simulink model "SPGF_FSK_0000_R2022b"  (R2022b)
settings: Solver=ode4  StartTime=0.0  StopTime=1.4  FixedStep=50e-6/50  RelTol=1e-3  EnableMultiTasking=on
undefined symbols (not defined in the file): D11, Delta
libraries: spsSeriesRLCBranchLib x1646, spsGroundLib x360, spsStairGeneratorLib x147, spsIdealSwitchLib x145, spsCurrentMeasurementLib x145, spsUniversalBridgeLib x76, spsThreePhaseSeriesRLCLoadLib x57, simulink x45, spsBistableLib x36, spsSequenceAnalyzerLib x31, spsThreePhaseParallelRLCLoadLib x20, spsThreePhaseTransformerTwoWindingsLib x20
(part 4 of 40)

== system SPGF_FSK_0000_R2022b/K6 ==
  fault : Subsystem  mask(Single Phase-to-Ground Fault){FaultA=on, FaultB=off, FaultC=off, FaultResistance=0.0001, GroundResistance=1e-03, SnubberResistance=1e6, SnubberCapacitance=inf, TransitionTimes=[0.2 0.8], InitialPhaseCtrl=off, Freq=50, Units=degrees, FaultDelayDeg=0, FaultDelayRad=0, FaultDelaySec=0, TheoryOfArc=None, WaitTime=0.008, TypeOfArcIgnVoltage=Stair Pattern with Ramp, ArcVoltage=6000, PulseArcVoltage=[6000 600], DurPulseArcVoltage=0.2, SwitchArcVoltage=[6000 600 5000 400], DurArcVoltage=[0.1 0.2 0.1 0.2], EndArcVoltage=[7000 200 5000 900], LimitArcNum=off, ArcingNumber=1, AddTimeDelay=off, TimeDelay=[0 0.1 0.2 ], EnableFilter=off, FreqFilter=200, FilterReturnTime=1e-3, Inter=off, TypeOfPause=None, NoiseSampleTime=0.04, NoiseSeed=23345, PulsePeriod=0.2, PulseWidth=20, PhaseDelay=0, SwitchTimes=[1 1.01 1.2 1.4]}
      mask prompts: FaultA "Phase A"; FaultB "Phase B"; FaultC "Phase C"; FaultResistance "Fault resistance Ron (ohms) :"; GroundResistance "Ground resistance Rg (ohms) :"; SnubberResistance "Snubbers resistance Rp (ohms) :"; SnubberCapacitance "Snubbers capacitance Cp (F) :"; TransitionTimes "Transition times (s) :"; InitialPhaseCtrl "Enable voltage zero crossing control"; Freq "Fundumental frequency (Hz) :"; Units "Units for fault delay"; FaultDelayDeg "Fault delay (Units) :"; FaultDelayRad "Fault delay (Units) :"; FaultDelaySec "Fault delay (Units) :"; TheoryOfArc "Theory of the arcing ground"; WaitTime "Wait time after the arcing (sec):"; TypeOfArcIgnVoltage "Type of Arc Ignition Voltage"; ArcVoltage "Voltage of the arcing (V) :"; PulseArcVoltage "Voltage of the arcing (V) :"; DurPulseArcVoltage "Duration of pulse (sec) :"; SwitchArcVoltage "Voltage of the arcing (V) :"; DurArcVoltage "Duration of Voltage Arc (sec) :"; EndArcVoltage "Voltage of the arcing at the end of each range (V) :"; LimitArcNum "Limit number of arcing [N] :"; ArcingNumber "Number of uprising arcing"; AddTimeDelay "Add time delay :"; TimeDelay "Time delay between arc (sec) [1xN] :"; EnableFilter "Enable lowpass filter"; FreqFilter "Natural frequency of lowpass filter (Hz) [120-250]:"; FilterReturnTime "Filter return time (sec):"; Inter "Interrupt only arc striking"; TypeOfPause "Add pause in the arcing ground"; NoiseSampleTime "Sample time of white noise (s) :"; NoiseSeed "Seed of white noise"; PulsePeriod "Period of pulses (s) :"; PulseWidth "Width of pulse (% of period) :"; PhaseDelay "Phase delay (sec) :"; SwitchTimes "Switch times (sec) [1,0,1,0...] :"
      mask init: same as SPGF_FSK_0000_R2022b/K2/fault
      settings: CloseFcn=|
      | en = get_param(gcb,'MaskEnables');
      | set_param(gcb,'MaskEnables',en)
      | clear enab en;
      settings: MoveFcn=|
      | en = get_param(gcb,'MaskEnables');
      | set_param(gcb,'MaskEnables',en)
      | clear enab en;
      mask Callback FaultA:
      | maskObj = Simulink.Mask.get(gcb);
      |     enab = get_param(gcb,'FaultA');
      |     if strcmp(enab,'on')
      |         maskObj.getParameter('FaultB').Enabled = 'off';
      |         maskObj.getParameter('FaultC').Enabled = 'off';
      |     else
      |         maskObj.getParameter('FaultB').Enabled = 'on';
      |         maskObj.getParameter('FaultC').Enabled = 'on';
      |     end
      mask Callback FaultB:
      | maskObj = Simulink.Mask.get(gcb);
      |     enab = get_param(gcb,'FaultB');
      |     if strcmp(enab,'on')
      |         maskObj.getParameter('FaultA').Enabled = 'off';
      |         maskObj.getParameter('FaultC').Enabled = 'off';
      |     else
      |         maskObj.getParameter('FaultA').Enabled = 'on';
      |         maskObj.getParameter('FaultC').Enabled = 'on';
      |     end
      mask Callback FaultC:
      | maskObj = Simulink.Mask.get(gcb);
      |     enab = get_param(gcb,'FaultC');
      |     if strcmp(enab,'on')
      |         maskObj.getParameter('FaultA').Enabled = 'off';
      |         maskObj.getParameter('FaultB').Enabled = 'off';
      |     else
      |         maskObj.getParameter('FaultA').Enabled = 'on';
      |         maskObj.getParameter('FaultB').Enabled = 'on';
      |     end
      mask Callback InitialPhaseCtrl:
      | maskObj = Simulink.Mask.get(gcb);
      |     enab = get_param(gcb,'InitialPhaseCtrl');
      |     units = get_param(gcb,'Units');
      |     if strcmp(enab,'on')
      |         maskObj.getParameter('Freq').Enabled = 'on';
      |         maskObj.getParameter('Units').Enabled = 'on';
      |         if strcmp(units,'degrees')
      |             maskObj.getParameter('FaultDelayDeg').Enabled = 'on';
      |         elseif strcmp(units,'radians')
      |             maskObj.getParameter('FaultDelayRad').Enabled = 'on';
      |         elseif strcmp(units,'seconds')
      |             maskObj.getParameter('FaultDelaySec').Enabled = 'on';
      |         end
      |     else
      |         maskObj.getParameter('Freq').Enabled = 'off';
      |         maskObj.getParameter('Units').Enabled = 'off';
      |         if strcmp(units,'degrees')
      |             maskObj.getParameter('FaultDelayDeg').Enabled = 'off';
      |         elseif strcmp(units,'radians')
      |             maskObj.getParameter('FaultDelayRad').Enabled = 'off';
      |         elseif strcmp(units,'seconds')
      |             maskObj.getParameter('FaultDelaySec').Enabled = 'off';
      |         end
      |     end
      mask TypeOptions Units: degrees | radians | seconds
      mask Callback Units:
      | maskObj = Simulink.Mask.get(gcb);
      |     units = get_param(gcb,'Units');
      |     if strcmp(units,'degrees')
      |         maskObj.getParameter('FaultDelayDeg').Visible = 'on';
      |         maskObj.getParameter('FaultDelayRad').Visible = 'off';
      |         maskObj.getParameter('FaultDelaySec').Visible = 'off';
      |     elseif strcmp(units,'radians')
      |         maskObj.getParameter('FaultDelayDeg').Visible = 'off';
      |         maskObj.getParameter('FaultDelayRad').Visible = 'on';
      |         maskObj.getParameter('FaultDelaySec').Visible = 'off';
      |     elseif strcmp(units,'seconds')
      |         maskObj.getParameter('FaultDelayDeg').Visible = 'off';
      |         maskObj.getParameter('FaultDelayRad').Visible = 'off';
      |         maskObj.getParameter('FaultDelaySec').Visible = 'on';
      |     end
      mask TypeOptions TheoryOfArc: None | Petersen | Peters & Slepian
      mask Callback TheoryOfArc:
      | maskObj = Simulink.Mask.get(gcb);
      |     param = get_param(gcb,'TheoryOfArc');
      |     if strcmp(param,'None')
      |         maskObj.getDialogControl('ContArcParam').Enabled = 'off';
      |     else
      |         maskObj.getDialogControl('ContArcParam').Enabled = 'on';
      |         if strcmp(param,'Peters & Slepian')
      |             maskObj.getDialogControl('ContFilterPetSlep').Visible = 'on';
      |             maskObj.getDialogControl('ContWaitPetSlep').Visible = 'on';
      |         else
      |             maskObj.getDialogControl('ContFilterPetSlep').Visible = 'off';
      |             maskObj.getDialogControl('ContWaitPetSlep').Visible = 'off';
      |         end
      |     end
      mask TypeOptions TypeOfArcIgnVoltage: Linear | Pulse Generator | Stair Pattern | Stair Pattern with Ramp
      mask Callback TypeOfArcIgnVoltage:
      | maskObj = Simulink.Mask.get(gcb);
      |     param = get_param(gcb,'TypeOfArcIgnVoltage');
      |     if strcmp(param,'Linear')
      |         maskObj.getParameter('ArcVoltage').Visible = 'on';
      |         maskObj.getParameter('PulseArcVoltage').Visible = 'off';
      |         maskObj.getParameter('DurPulseArcVoltage').Visible = 'off';
      |         maskObj.getParameter('SwitchArcVoltage').Visible = 'off';
      |         maskObj.getParameter('DurArcVoltage').Visible = 'off';
      |         maskObj.getParameter('EndArcVoltage').Visible = 'off';
      |     elseif strcmp(param,'Pulse Generator')
      |         maskObj.getParameter('ArcVoltage').Visible = 'off';
      |         maskObj.getParameter('PulseArcVoltage').Visible = 'on';
      |         maskObj.getParameter('DurPulseArcVoltage').Visible = 'on';
      |         maskObj.getParameter('SwitchArcVoltage').Visible = 'off';
      |         maskObj.getParameter('DurArcVoltage').Visible = 'off';
      |         maskObj.getParameter('EndArcVoltage').Visible = 'off';
      |     elseif strcmp(param,'Stair Pattern')
      |         maskObj.getParameter('ArcVoltage').Visible = 'off';
      |         maskObj.getParameter('PulseArcVoltage').Visible = 'off';
      |         maskObj.getParameter('DurPulseArcVoltage').Visible = 'off';
      |         maskObj.getParameter('SwitchArcVoltage').Visible = 'on';
      |         maskObj.getParameter('DurArcVoltage').Visible = 'on';
      |         maskObj.getParameter('EndArcVoltage').Visible = 'off';
      |     elseif strcmp(param,'Stair Pattern with Ramp')
      |         maskObj.getParameter('ArcVoltage').Visible = 'off';
      |         maskObj.getParameter('PulseArcVoltage').Visible = 'off';
      |         maskObj.getParameter('DurPulseArcVoltage').Visible = 'off';
      |         maskObj.getParameter('SwitchArcVoltage').Visible = 'on';
      |         maskObj.getParameter('DurArcVoltage').Visible = 'on';
      |         maskObj.getParameter('EndArcVoltage').Visible = 'on';
      |     end
      mask Callback LimitArcNum:
      | maskObj = Simulink.Mask.get(gcb);
      |     enab = get_param(gcb,'LimitArcNum');
      |     if strcmp(enab,'on')
      |         maskObj.getParameter('ArcingNumber').Visible = 'on';
      |         maskObj.getParameter('AddTimeDelay').Visible = 'on';
      |     else
      |         maskObj.getParameter('ArcingNumber').Visible = 'off';
      |         set_param(gcb,'AddTimeDelay','off');
      |         maskObj.getParameter('AddTimeDelay').Visible = 'off';
      |         maskObj.getParameter('TimeDelay').Visible = 'off';
      |     end
      mask Callback AddTimeDelay:
      | maskObj = Simulink.Mask.get(gcb);
      |     enab = get_param(gcb,'AddTimeDelay');
      |     if strcmp(enab,'on')
      |         maskObj.getParameter('TimeDelay').Visible = 'on';
      |     else
      |         maskObj.getParameter('TimeDelay').Visible = 'off';
      |     end
      mask Callback EnableFilter:
      | maskObj = Simulink.Mask.get(gcb);
      |     enab = get_param(gcb,'EnableFilter');
      |     if strcmp(enab,'on')
      |         maskObj.getParameter('FreqFilter').Visible = 'on';
      |         maskObj.getParameter('FilterReturnTime').Visible = 'on';
      |     else
      |         maskObj.getParameter('FreqFilter').Visible = 'off';
      |         maskObj.getParameter('FilterReturnTime').Visible = 'off';
      |     end
      mask TypeOptions TypeOfPause: None | White Noise | Pulse Generator | Time Dependent Pulses
      mask Callback TypeOfPause:
      | maskObj = Simulink.Mask.get(gcb);
      |     enab = get_param(gcb,'TypeOfPause');
      |     if strcmp(enab,'None')
      |         maskObj.getParameter('NoiseSampleTime').Visible = 'off';
      |         maskObj.getParameter('NoiseSeed').Visible = 'off';
      |         maskObj.getParameter('PulsePeriod').Visible = 'off';
      |         maskObj.getParameter('PulseWidth').Visible = 'off';
      |         maskObj.getParameter('PhaseDelay').Visible = 'off';
      |         maskObj.getParameter('SwitchTimes').Visible = 'off';
      |     elseif strcmp(enab,'White Noise')
      |         maskObj.getParameter('NoiseSampleTime').Visible = 'on';
      |         maskObj.getParameter('NoiseSeed').Visible = 'on';
      |         maskObj.getParameter('PulsePeriod').Visible = 'off';
      |         maskObj.getParameter('PulseWidth').Visible = 'off';
      |         maskObj.getParameter('PhaseDelay').Visible = 'off';
      |         maskObj.getParameter('SwitchTimes').Visible = 'off';
      |     elseif strcmp(enab,'Pulse Generator')
      |         maskObj.getParameter('NoiseSampleTime').Visible = 'off';
      |         maskObj.getParameter('NoiseSeed').Visible = 'off';
      |         maskObj.getParameter('PulsePeriod').Visible = 'on';
      |         maskObj.getParameter('PulseWidth').Visible = 'on';
      |         maskObj.getParameter('PhaseDelay').Visible = 'on';
      |         maskObj.getParameter('SwitchTimes').Visible = 'off';
      |     elseif strcmp(enab,'Time Dependent Pulses')
      |         maskObj.getParameter('NoiseSampleTime').Visible = 'off';
      |         maskObj.getParameter('NoiseSeed').Visible = 'off';
      |         maskObj.getParameter('PulsePeriod').Visible = 'off';
      |         maskObj.getParameter('PulseWidth').Visible = 'off';
      |         maskObj.getParameter('PhaseDelay').Visible = 'off';
      |         maskObj.getParameter('SwitchTimes').Visible = 'on';
      |     end
      mask DialogControl Container4 Prompt: Configuration
      mask DialogControl ContFaultABC Prompt: Fault :
      mask DialogControl ContBreakerParam Prompt: Breaker parameters :
      mask DialogControl ContZeroCross Prompt: Control initial voltage phase of first fault
      mask DialogControl Container5 Prompt: Arc Parameters
      mask DialogControl ContArcParam Prompt: Arc fault parameters
      mask DialogControl ContArcVoltage Prompt: Arc Ignition Voltage
      mask DialogControl ContArcLim Prompt: Arc limitations
      mask DialogControl ContFilterPetSlep Prompt: Filtering
      mask DialogControl ContInterruption Prompt: Interruption
      mask DialogControl Container14 Prompt: Settings for different types of fault interruption
      mask Display:
      | % port_label('input',1,'Iabc');
      | 
      | port_label('lconn',1,'A');
      | port_label('lconn',2,'B');
      | port_label('lconn',3,'C');
      | 
      | disp('   SPGF    ');
  meas : Subsystem
  A : PMIOPort  Side=Left
  B : PMIOPort  Port=2  Side=Left
  C : PMIOPort  Port=3  Side=Left
  connections:
  fault/LConn1 -- meas/RConn1
  fault/LConn2 -- meas/RConn2
  fault/LConn3 -- meas/RConn3
  meas/LConn2 -- B/RConn1
  meas/LConn1 -- A/RConn1
  meas/LConn3 -- C/RConn1

== system SPGF_FSK_0000_R2022b/K8 ==
  fault : Subsystem  mask(Single Phase-to-Ground Fault){FaultA=on, FaultB=off, FaultC=off, FaultResistance=0.0001, GroundResistance=1e-03, SnubberResistance=1e6, SnubberCapacitance=inf, TransitionTimes=[0.2 0.8], InitialPhaseCtrl=off, Freq=50, Units=degrees, FaultDelayDeg=0, FaultDelayRad=0, FaultDelaySec=0, TheoryOfArc=None, WaitTime=0.008, TypeOfArcIgnVoltage=Stair Pattern with Ramp, ArcVoltage=6000, PulseArcVoltage=[6000 600], DurPulseArcVoltage=0.2, SwitchArcVoltage=[6000 600 5000 400], DurArcVoltage=[0.1 0.2 0.1 0.2], EndArcVoltage=[7000 200 5000 900], LimitArcNum=off, ArcingNumber=1, AddTimeDelay=off, TimeDelay=[0 0.1 0.2 ], EnableFilter=off, FreqFilter=200, FilterReturnTime=1e-3, Inter=off, TypeOfPause=None, NoiseSampleTime=0.04, NoiseSeed=23345, PulsePeriod=0.2, PulseWidth=20, PhaseDelay=0, SwitchTimes=[1 1.01 1.2 1.4]}
      mask prompts: FaultA "Phase A"; FaultB "Phase B"; FaultC "Phase C"; FaultResistance "Fault resistance Ron (ohms) :"; GroundResistance "Ground resistance Rg (ohms) :"; SnubberResistance "Snubbers resistance Rp (ohms) :"; SnubberCapacitance "Snubbers capacitance Cp (F) :"; TransitionTimes "Transition times (s) :"; InitialPhaseCtrl "Enable voltage zero crossing control"; Freq "Fundumental frequency (Hz) :"; Units "Units for fault delay"; FaultDelayDeg "Fault delay (Units) :"; FaultDelayRad "Fault delay (Units) :"; FaultDelaySec "Fault delay (Units) :"; TheoryOfArc "Theory of the arcing ground"; WaitTime "Wait time after the arcing (sec):"; TypeOfArcIgnVoltage "Type of Arc Ignition Voltage"; ArcVoltage "Voltage of the arcing (V) :"; PulseArcVoltage "Voltage of the arcing (V) :"; DurPulseArcVoltage "Duration of pulse (sec) :"; SwitchArcVoltage "Voltage of the arcing (V) :"; DurArcVoltage "Duration of Voltage Arc (sec) :"; EndArcVoltage "Voltage of the arcing at the end of each range (V) :"; LimitArcNum "Limit number of arcing [N] :"; ArcingNumber "Number of uprising arcing"; AddTimeDelay "Add time delay :"; TimeDelay "Time delay between arc (sec) [1xN] :"; EnableFilter "Enable lowpass filter"; FreqFilter "Natural frequency of lowpass filter (Hz) [120-250]:"; FilterReturnTime "Filter return time (sec):"; Inter "Interrupt only arc striking"; TypeOfPause "Add pause in the arcing ground"; NoiseSampleTime "Sample time of white noise (s) :"; NoiseSeed "Seed of white noise"; PulsePeriod "Period of pulses (s) :"; PulseWidth "Width of pulse (% of period) :"; PhaseDelay "Phase delay (sec) :"; SwitchTimes "Switch times (sec) [1,0,1,0...] :"
      mask init: same as SPGF_FSK_0000_R2022b/K2/fault
      settings: CloseFcn=|
      | en = get_param(gcb,'MaskEnables');
      | set_param(gcb,'MaskEnables',en)
      | clear enab en;
      settings: MoveFcn=|
      | en = get_param(gcb,'MaskEnables');
      | set_param(gcb,'MaskEnables',en)
      | clear enab en;
      mask Callback FaultA:
      | maskObj = Simulink.Mask.get(gcb);
      |     enab = get_param(gcb,'FaultA');
      |     if strcmp(enab,'on')
      |         maskObj.getParameter('FaultB').Enabled = 'off';
      |         maskObj.getParameter('FaultC').Enabled = 'off';
      |     else
      |         maskObj.getParameter('FaultB').Enabled = 'on';
      |         maskObj.getParameter('FaultC').Enabled = 'on';
      |     end
      mask Callback FaultB:
      | maskObj = Simulink.Mask.get(gcb);
      |     enab = get_param(gcb,'FaultB');
      |     if strcmp(enab,'on')
      |         maskObj.getParameter('FaultA').Enabled = 'off';
      |         maskObj.getParameter('FaultC').Enabled = 'off';
      |     else
      |         maskObj.getParameter('FaultA').Enabled = 'on';
      |         maskObj.getParameter('FaultC').Enabled = 'on';
      |     end
      mask Callback FaultC:
      | maskObj = Simulink.Mask.get(gcb);
      |     enab = get_param(gcb,'FaultC');
      |     if strcmp(enab,'on')
      |         maskObj.getParameter('FaultA').Enabled = 'off';
      |         maskObj.getParameter('FaultB').Enabled = 'off';
      |     else
      |         maskObj.getParameter('FaultA').Enabled = 'on';
      |         maskObj.getParameter('FaultB').Enabled = 'on';
      |     end
      mask Callback InitialPhaseCtrl:
      | maskObj = Simulink.Mask.get(gcb);
      |     enab = get_param(gcb,'InitialPhaseCtrl');
      |     units = get_param(gcb,'Units');
      |     if strcmp(enab,'on')
      |         maskObj.getParameter('Freq').Enabled = 'on';
      |         maskObj.getParameter('Units').Enabled = 'on';
      |         if strcmp(units,'degrees')
      |             maskObj.getParameter('FaultDelayDeg').Enabled = 'on';
      |         elseif strcmp(units,'radians')
      |             maskObj.getParameter('FaultDelayRad').Enabled = 'on';
      |         elseif strcmp(units,'seconds')
      |             maskObj.getParameter('FaultDelaySec').Enabled = 'on';
      |         end
      |     else
      |         maskObj.getParameter('Freq').Enabled = 'off';
      |         maskObj.getParameter('Units').Enabled = 'off';
      |         if strcmp(units,'degrees')
      |             maskObj.getParameter('FaultDelayDeg').Enabled = 'off';
      |         elseif strcmp(units,'radians')
      |             maskObj.getParameter('FaultDelayRad').Enabled = 'off';
      |         elseif strcmp(units,'seconds')
      |             maskObj.getParameter('FaultDelaySec').Enabled = 'off';
      |         end
      |     end
      mask TypeOptions Units: degrees | radians | seconds
      mask Callback Units:
      | maskObj = Simulink.Mask.get(gcb);
      |     units = get_param(gcb,'Units');
      |     if strcmp(units,'degrees')
      |         maskObj.getParameter('FaultDelayDeg').Visible = 'on';
      |         maskObj.getParameter('FaultDelayRad').Visible = 'off';
      |         maskObj.getParameter('FaultDelaySec').Visible = 'off';
      |     elseif strcmp(units,'radians')
      |         maskObj.getParameter('FaultDelayDeg').Visible = 'off';
      |         maskObj.getParameter('FaultDelayRad').Visible = 'on';
      |         maskObj.getParameter('FaultDelaySec').Visible = 'off';
      |     elseif strcmp(units,'seconds')
      |         maskObj.getParameter('FaultDelayDeg').Visible = 'off';
      |         maskObj.getParameter('FaultDelayRad').Visible = 'off';
      |         maskObj.getParameter('FaultDelaySec').Visible = 'on';
      |     end
      mask TypeOptions TheoryOfArc: None | Petersen | Peters & Slepian
      mask Callback TheoryOfArc:
      | maskObj = Simulink.Mask.get(gcb);
      |     param = get_param(gcb,'TheoryOfArc');
      |     if strcmp(param,'None')
      |         maskObj.getDialogControl('ContArcParam').Enabled = 'off';
      |     else
      |         maskObj.getDialogControl('ContArcParam').Enabled = 'on';
      |         if strcmp(param,'Peters & Slepian')
      |             maskObj.getDialogControl('ContFilterPetSlep').Visible = 'on';
      |             maskObj.getDialogControl('ContWaitPetSlep').Visible = 'on';
      |         else
      |             maskObj.getDialogControl('ContFilterPetSlep').Visible = 'off';
      |             maskObj.getDialogControl('ContWaitPetSlep').Visible = 'off';
      |         end
      |     end
      mask TypeOptions TypeOfArcIgnVoltage: Linear | Pulse Generator | Stair Pattern | Stair Pattern with Ramp
      mask Callback TypeOfArcIgnVoltage:
      | maskObj = Simulink.Mask.get(gcb);
      |     param = get_param(gcb,'TypeOfArcIgnVoltage');
      |     if strcmp(param,'Linear')
      |         maskObj.getParameter('ArcVoltage').Visible = 'on';
      |         maskObj.getParameter('PulseArcVoltage').Visible = 'off';
      |         maskObj.getParameter('DurPulseArcVoltage').Visible = 'off';
      |         maskObj.getParameter('SwitchArcVoltage').Visible = 'off';
      |         maskObj.getParameter('DurArcVoltage').Visible = 'off';
      |         maskObj.getParameter('EndArcVoltage').Visible = 'off';
      |     elseif strcmp(param,'Pulse Generator')
      |         maskObj.getParameter('ArcVoltage').Visible = 'off';
      |         maskObj.getParameter('PulseArcVoltage').Visible = 'on';
      |         maskObj.getParameter('DurPulseArcVoltage').Visible = 'on';
      |         maskObj.getParameter('SwitchArcVoltage').Visible = 'off';
      |         maskObj.getParameter('DurArcVoltage').Visible = 'off';
      |         maskObj.getParameter('EndArcVoltage').Visible = 'off';
      |     elseif strcmp(param,'Stair Pattern')
      |         maskObj.getParameter('ArcVoltage').Visible = 'off';
      |         maskObj.getParameter('PulseArcVoltage').Visible = 'off';
      |         maskObj.getParameter('DurPulseArcVoltage').Visible = 'off';
      |         maskObj.getParameter('SwitchArcVoltage').Visible = 'on';
      |         maskObj.getParameter('DurArcVoltage').Visible = 'on';
      |         maskObj.getParameter('EndArcVoltage').Visible = 'off';
      |     elseif strcmp(param,'Stair Pattern with Ramp')
      |         maskObj.getParameter('ArcVoltage').Visible = 'off';
      |         maskObj.getParameter('PulseArcVoltage').Visible = 'off';
      |         maskObj.getParameter('DurPulseArcVoltage').Visible = 'off';
      |         maskObj.getParameter('SwitchArcVoltage').Visible = 'on';
      |         maskObj.getParameter('DurArcVoltage').Visible = 'on';
      |         maskObj.getParameter('EndArcVoltage').Visible = 'on';
      |     end
      mask Callback LimitArcNum:
      | maskObj = Simulink.Mask.get(gcb);
      |     enab = get_param(gcb,'LimitArcNum');
      |     if strcmp(enab,'on')
      |         maskObj.getParameter('ArcingNumber').Visible = 'on';
      |         maskObj.getParameter('AddTimeDelay').Visible = 'on';
      |     else
      |         maskObj.getParameter('ArcingNumber').Visible = 'off';
      |         set_param(gcb,'AddTimeDelay','off');
      |         maskObj.getParameter('AddTimeDelay').Visible = 'off';
      |         maskObj.getParameter('TimeDelay').Visible = 'off';
      |     end
      mask Callback AddTimeDelay:
      | maskObj = Simulink.Mask.get(gcb);
      |     enab = get_param(gcb,'AddTimeDelay');
      |     if strcmp(enab,'on')
      |         maskObj.getParameter('TimeDelay').Visible = 'on';
      |     else
      |         maskObj.getParameter('TimeDelay').Visible = 'off';
      |     end
      mask Callback EnableFilter:
      | maskObj = Simulink.Mask.get(gcb);
      |     enab = get_param(gcb,'EnableFilter');
      |     if strcmp(enab,'on')
      |         maskObj.getParameter('FreqFilter').Visible = 'on';
      |         maskObj.getParameter('FilterReturnTime').Visible = 'on';
      |     else
      |         maskObj.getParameter('FreqFilter').Visible = 'off';
      |         maskObj.getParameter('FilterReturnTime').Visible = 'off';
      |     end
      mask TypeOptions TypeOfPause: None | White Noise | Pulse Generator | Time Dependent Pulses
      mask Callback TypeOfPause:
      | maskObj = Simulink.Mask.get(gcb);
      |     enab = get_param(gcb,'TypeOfPause');
      |     if strcmp(enab,'None')
      |         maskObj.getParameter('NoiseSampleTime').Visible = 'off';
      |         maskObj.getParameter('NoiseSeed').Visible = 'off';
      |         maskObj.getParameter('PulsePeriod').Visible = 'off';
      |         maskObj.getParameter('PulseWidth').Visible = 'off';
      |         maskObj.getParameter('PhaseDelay').Visible = 'off';
      |         maskObj.getParameter('SwitchTimes').Visible = 'off';
      |     elseif strcmp(enab,'White Noise')
      |         maskObj.getParameter('NoiseSampleTime').Visible = 'on';
      |         maskObj.getParameter('NoiseSeed').Visible = 'on';
      |         maskObj.getParameter('PulsePeriod').Visible = 'off';
      |         maskObj.getParameter('PulseWidth').Visible = 'off';
      |         maskObj.getParameter('PhaseDelay').Visible = 'off';
      |         maskObj.getParameter('SwitchTimes').Visible = 'off';
      |     elseif strcmp(enab,'Pulse Generator')
      |         maskObj.getParameter('NoiseSampleTime').Visible = 'off';
      |         maskObj.getParameter('NoiseSeed').Visible = 'off';
      |         maskObj.getParameter('PulsePeriod').Visible = 'on';
      |         maskObj.getParameter('PulseWidth').Visible = 'on';
      |         maskObj.getParameter('PhaseDelay').Visible = 'on';
      |         maskObj.getParameter('SwitchTimes').Visible = 'off';
      |     elseif strcmp(enab,'Time Dependent Pulses')
      |         maskObj.getParameter('NoiseSampleTime').Visible = 'off';
      |         maskObj.getParameter('NoiseSeed').Visible = 'off';
      |         maskObj.getParameter('PulsePeriod').Visible = 'off';
      |         maskObj.getParameter('PulseWidth').Visible = 'off';
      |         maskObj.getParameter('PhaseDelay').Visible = 'off';
      |         maskObj.getParameter('SwitchTimes').Visible = 'on';
      |     end
      mask DialogControl Container4 Prompt: Configuration
      mask DialogControl ContFaultABC Prompt: Fault :
      mask DialogControl ContBreakerParam Prompt: Breaker parameters :
      mask DialogControl ContZeroCross Prompt: Control initial voltage phase of first fault
      mask DialogControl Container5 Prompt: Arc Parameters
      mask DialogControl ContArcParam Prompt: Arc fault parameters
      mask DialogControl ContArcVoltage Prompt: Arc Ignition Voltage
      mask DialogControl ContArcLim Prompt: Arc limitations
      mask DialogControl ContFilterPetSlep Prompt: Filtering
      mask DialogControl ContInterruption Prompt: Interruption
      mask DialogControl Container14 Prompt: Settings for different types of fault interruption
      mask Display:
      | % port_label('input',1,'Iabc');
      | 
      | port_label('lconn',1,'A');
      | port_label('lconn',2,'B');
      | port_label('lconn',3,'C');
      | 
      | disp('   SPGF    ');
  meas : Subsystem
  A : PMIOPort  Side=Left
  B : PMIOPort  Port=2  Side=Left
  C : PMIOPort  Port=3  Side=Left
  connections:
  fault/LConn1 -- meas/RConn1
  fault/LConn2 -- meas/RConn2
  fault/LConn3 -- meas/RConn3
  meas/LConn2 -- B/RConn1
  meas/LConn1 -- A/RConn1
  meas/LConn3 -- C/RConn1

== system SPGF_FSK_0000_R2022b/K9 ==
  fault : Subsystem  mask(Single Phase-to-Ground Fault){FaultA=on, FaultB=off, FaultC=off, FaultResistance=0.0001, GroundResistance=1e-03, SnubberResistance=1e6, SnubberCapacitance=inf, TransitionTimes=[0.2 0.8], InitialPhaseCtrl=off, Freq=50, Units=degrees, FaultDelayDeg=0, FaultDelayRad=0, FaultDelaySec=0, TheoryOfArc=None, WaitTime=0.008, TypeOfArcIgnVoltage=Stair Pattern with Ramp, ArcVoltage=6000, PulseArcVoltage=[6000 600], DurPulseArcVoltage=0.2, SwitchArcVoltage=[6000 600 5000 400], DurArcVoltage=[0.1 0.2 0.1 0.2], EndArcVoltage=[7000 200 5000 900], LimitArcNum=off, ArcingNumber=1, AddTimeDelay=off, TimeDelay=[0 0.1 0.2 ], EnableFilter=off, FreqFilter=200, FilterReturnTime=1e-3, Inter=off, TypeOfPause=None, NoiseSampleTime=0.04, NoiseSeed=23345, PulsePeriod=0.2, PulseWidth=20, PhaseDelay=0, SwitchTimes=[1 1.01 1.2 1.4]}
      mask prompts: FaultA "Phase A"; FaultB "Phase B"; FaultC "Phase C"; FaultResistance "Fault resistance Ron (ohms) :"; GroundResistance "Ground resistance Rg (ohms) :"; SnubberResistance "Snubbers resistance Rp (ohms) :"; SnubberCapacitance "Snubbers capacitance Cp (F) :"; TransitionTimes "Transition times (s) :"; InitialPhaseCtrl "Enable voltage zero crossing control"; Freq "Fundumental frequency (Hz) :"; Units "Units for fault delay"; FaultDelayDeg "Fault delay (Units) :"; FaultDelayRad "Fault delay (Units) :"; FaultDelaySec "Fault delay (Units) :"; TheoryOfArc "Theory of the arcing ground"; WaitTime "Wait time after the arcing (sec):"; TypeOfArcIgnVoltage "Type of Arc Ignition Voltage"; ArcVoltage "Voltage of the arcing (V) :"; PulseArcVoltage "Voltage of the arcing (V) :"; DurPulseArcVoltage "Duration of pulse (sec) :"; SwitchArcVoltage "Voltage of the arcing (V) :"; DurArcVoltage "Duration of Voltage Arc (sec) :"; EndArcVoltage "Voltage of the arcing at the end of each range (V) :"; LimitArcNum "Limit number of arcing [N] :"; ArcingNumber "Number of uprising arcing"; AddTimeDelay "Add time delay :"; TimeDelay "Time delay between arc (sec) [1xN] :"; EnableFilter "Enable lowpass filter"; FreqFilter "Natural frequency of lowpass filter (Hz) [120-250]:"; FilterReturnTime "Filter return time (sec):"; Inter "Interrupt only arc striking"; TypeOfPause "Add pause in the arcing ground"; NoiseSampleTime "Sample time of white noise (s) :"; NoiseSeed "Seed of white noise"; PulsePeriod "Period of pulses (s) :"; PulseWidth "Width of pulse (% of period) :"; PhaseDelay "Phase delay (sec) :"; SwitchTimes "Switch times (sec) [1,0,1,0...] :"
      mask init: same as SPGF_FSK_0000_R2022b/K2/fault
      settings: CloseFcn=|
      | en = get_param(gcb,'MaskEnables');
      | set_param(gcb,'MaskEnables',en)
      | clear enab en;
      settings: MoveFcn=|
      | en = get_param(gcb,'MaskEnables');
      | set_param(gcb,'MaskEnables',en)
      | clear enab en;
      mask Callback FaultA:
      | maskObj = Simulink.Mask.get(gcb);
      |     enab = get_param(gcb,'FaultA');
      |     if strcmp(enab,'on')
      |         maskObj.getParameter('FaultB').Enabled = 'off';
      |         maskObj.getParameter('FaultC').Enabled = 'off';
      |     else
      |         maskObj.getParameter('FaultB').Enabled = 'on';
      |         maskObj.getParameter('FaultC').Enabled = 'on';
      |     end
      mask Callback FaultB:
      | maskObj = Simulink.Mask.get(gcb);
      |     enab = get_param(gcb,'FaultB');
      |     if strcmp(enab,'on')
      |         maskObj.getParameter('FaultA').Enabled = 'off';
      |         maskObj.getParameter('FaultC').Enabled = 'off';
      |     else
      |         maskObj.getParameter('FaultA').Enabled = 'on';
      |         maskObj.getParameter('FaultC').Enabled = 'on';
      |     end
      mask Callback FaultC:
      | maskObj = Simulink.Mask.get(gcb);
      |     enab = get_param(gcb,'FaultC');
      |     if strcmp(enab,'on')
      |         maskObj.getParameter('FaultA').Enabled = 'off';
      |         maskObj.getParameter('FaultB').Enabled = 'off';
      |     else
      |         maskObj.getParameter('FaultA').Enabled = 'on';
      |         maskObj.getParameter('FaultB').Enabled = 'on';
      |     end
      mask Callback InitialPhaseCtrl:
      | maskObj = Simulink.Mask.get(gcb);
      |     enab = get_param(gcb,'InitialPhaseCtrl');
      |     units = get_param(gcb,'Units');
      |     if strcmp(enab,'on')
      |         maskObj.getParameter('Freq').Enabled = 'on';
      |         maskObj.getParameter('Units').Enabled = 'on';
      |         if strcmp(units,'degrees')
      |             maskObj.getParameter('FaultDelayDeg').Enabled = 'on';
      |         elseif strcmp(units,'radians')
      |             maskObj.getParameter('FaultDelayRad').Enabled = 'on';
      |         elseif strcmp(units,'seconds')
      |             maskObj.getParameter('FaultDelaySec').Enabled = 'on';
      |         end
      |     else
      |         maskObj.getParameter('Freq').Enabled = 'off';
      |         maskObj.getParameter('Units').Enabled = 'off';
      |         if strcmp(units,'degrees')
      |             maskObj.getParameter('FaultDelayDeg').Enabled = 'off';
      |         elseif strcmp(units,'radians')
      |             maskObj.getParameter('FaultDelayRad').Enabled = 'off';
      |         elseif strcmp(units,'seconds')
      |             maskObj.getParameter('FaultDelaySec').Enabled = 'off';
      |         end
      |     end
      mask TypeOptions Units: degrees | radians | seconds
      mask Callback Units:
      | maskObj = Simulink.Mask.get(gcb);
      |     units = get_param(gcb,'Units');
      |     if strcmp(units,'degrees')
      |         maskObj.getParameter('FaultDelayDeg').Visible = 'on';
      |         maskObj.getParameter('FaultDelayRad').Visible = 'off';
      |         maskObj.getParameter('FaultDelaySec').Visible = 'off';
      |     elseif strcmp(units,'radians')
      |         maskObj.getParameter('FaultDelayDeg').Visible = 'off';
      |         maskObj.getParameter('FaultDelayRad').Visible = 'on';
      |         maskObj.getParameter('FaultDelaySec').Visible = 'off';
      |     elseif strcmp(units,'seconds')
      |         maskObj.getParameter('FaultDelayDeg').Visible = 'off';
      |         maskObj.getParameter('FaultDelayRad').Visible = 'off';
      |         maskObj.getParameter('FaultDelaySec').Visible = 'on';
      |     end
      mask TypeOptions TheoryOfArc: None | Petersen | Peters & Slepian
      mask Callback TheoryOfArc:
      | maskObj = Simulink.Mask.get(gcb);
      |     param = get_param(gcb,'TheoryOfArc');
      |     if strcmp(param,'None')
      |         maskObj.getDialogControl('ContArcParam').Enabled = 'off';
      |     else
      |         maskObj.getDialogControl('ContArcParam').Enabled = 'on';
      |         if strcmp(param,'Peters & Slepian')
      |             maskObj.getDialogControl('ContFilterPetSlep').Visible = 'on';
      |             maskObj.getDialogControl('ContWaitPetSlep').Visible = 'on';
      |         else
      |             maskObj.getDialogControl('ContFilterPetSlep').Visible = 'off';
      |             maskObj.getDialogControl('ContWaitPetSlep').Visible = 'off';
      |         end
      |     end
      mask TypeOptions TypeOfArcIgnVoltage: Linear | Pulse Generator | Stair Pattern | Stair Pattern with Ramp
      mask Callback TypeOfArcIgnVoltage:
      | maskObj = Simulink.Mask.get(gcb);
      |     param = get_param(gcb,'TypeOfArcIgnVoltage');
      |     if strcmp(param,'Linear')
      |         maskObj.getParameter('ArcVoltage').Visible = 'on';
      |         maskObj.getParameter('PulseArcVoltage').Visible = 'off';
      |         maskObj.getParameter('DurPulseArcVoltage').Visible = 'off';
      |         maskObj.getParameter('SwitchArcVoltage').Visible = 'off';
      |         maskObj.getParameter('DurArcVoltage').Visible = 'off';
      |         maskObj.getParameter('EndArcVoltage').Visible = 'off';
      |     elseif strcmp(param,'Pulse Generator')
      |         maskObj.getParameter('ArcVoltage').Visible = 'off';
      |         maskObj.getParameter('PulseArcVoltage').Visible = 'on';
      |         maskObj.getParameter('DurPulseArcVoltage').Visible = 'on';
      |         maskObj.getParameter('SwitchArcVoltage').Visible = 'off';
      |         maskObj.getParameter('DurArcVoltage').Visible = 'off';
      |         maskObj.getParameter('EndArcVoltage').Visible = 'off';
      |     elseif strcmp(param,'Stair Pattern')
      |         maskObj.getParameter('ArcVoltage').Visible = 'off';
      |         maskObj.getParameter('PulseArcVoltage').Visible = 'off';
      |         maskObj.getParameter('DurPulseArcVoltage').Visible = 'off';
      |         maskObj.getParameter('SwitchArcVoltage').Visible = 'on';
      |         maskObj.getParameter('DurArcVoltage').Visible = 'on';
      |         maskObj.getParameter('EndArcVoltage').Visible = 'off';
      |     elseif strcmp(param,'Stair Pattern with Ramp')
      |         maskObj.getParameter('ArcVoltage').Visible = 'off';
      |         maskObj.getParameter('PulseArcVoltage').Visible = 'off';
      |         maskObj.getParameter('DurPulseArcVoltage').Visible = 'off';
      |         maskObj.getParameter('SwitchArcVoltage').Visible = 'on';
      |         maskObj.getParameter('DurArcVoltage').Visible = 'on';
      |         maskObj.getParameter('EndArcVoltage').Visible = 'on';
      |     end
      mask Callback LimitArcNum:
      | maskObj = Simulink.Mask.get(gcb);
      |     enab = get_param(gcb,'LimitArcNum');
      |     if strcmp(enab,'on')
      |         maskObj.getParameter('ArcingNumber').Visible = 'on';
      |         maskObj.getParameter('AddTimeDelay').Visible = 'on';
      |     else
      |         maskObj.getParameter('ArcingNumber').Visible = 'off';
      |         set_param(gcb,'AddTimeDelay','off');
      |         maskObj.getParameter('AddTimeDelay').Visible = 'off';
      |         maskObj.getParameter('TimeDelay').Visible = 'off';
      |     end
      mask Callback AddTimeDelay:
      | maskObj = Simulink.Mask.get(gcb);
      |     enab = get_param(gcb,'AddTimeDelay');
      |     if strcmp(enab,'on')
      |         maskObj.getParameter('TimeDelay').Visible = 'on';
      |     else
      |         maskObj.getParameter('TimeDelay').Visible = 'off';
      |     end
      mask Callback EnableFilter:
      | maskObj = Simulink.Mask.get(gcb);
      |     enab = get_param(gcb,'EnableFilter');
      |     if strcmp(enab,'on')
      |         maskObj.getParameter('FreqFilter').Visible = 'on';
      |         maskObj.getParameter('FilterReturnTime').Visible = 'on';
      |     else
      |         maskObj.getParameter('FreqFilter').Visible = 'off';
      |         maskObj.getParameter('FilterReturnTime').Visible = 'off';
      |     end
      mask TypeOptions TypeOfPause: None | White Noise | Pulse Generator | Time Dependent Pulses
      mask Callback TypeOfPause:
      | maskObj = Simulink.Mask.get(gcb);
      |     enab = get_param(gcb,'TypeOfPause');
      |     if strcmp(enab,'None')
      |         maskObj.getParameter('NoiseSampleTime').Visible = 'off';
      |         maskObj.getParameter('NoiseSeed').Visible = 'off';
      |         maskObj.getParameter('PulsePeriod').Visible = 'off';
      |         maskObj.getParameter('PulseWidth').Visible = 'off';
      |         maskObj.getParameter('PhaseDelay').Visible = 'off';
      |         maskObj.getParameter('SwitchTimes').Visible = 'off';
      |     elseif strcmp(enab,'White Noise')
      |         maskObj.getParameter('NoiseSampleTime').Visible = 'on';
      |         maskObj.getParameter('NoiseSeed').Visible = 'on';
      |         maskObj.getParameter('PulsePeriod').Visible = 'off';
      |         maskObj.getParameter('PulseWidth').Visible = 'off';
      |         maskObj.getParameter('PhaseDelay').Visible = 'off';
      |         maskObj.getParameter('SwitchTimes').Visible = 'off';
      |     elseif strcmp(enab,'Pulse Generator')
      |         maskObj.getParameter('NoiseSampleTime').Visible = 'off';
      |         maskObj.getParameter('NoiseSeed').Visible = 'off';
      |         maskObj.getParameter('PulsePeriod').Visible = 'on';
      |         maskObj.getParameter('PulseWidth').Visible = 'on';
      |         maskObj.getParameter('PhaseDelay').Visible = 'on';
      |         maskObj.getParameter('SwitchTimes').Visible = 'off';
      |     elseif strcmp(enab,'Time Dependent Pulses')
      |         maskObj.getParameter('NoiseSampleTime').Visible = 'off';
      |         maskObj.getParameter('NoiseSeed').Visible = 'off';
      |         maskObj.getParameter('PulsePeriod').Visible = 'off';
      |         maskObj.getParameter('PulseWidth').Visible = 'off';
      |         maskObj.getParameter('PhaseDelay').Visible = 'off';
      |         maskObj.getParameter('SwitchTimes').Visible = 'on';
      |     end
      mask DialogControl Container4 Prompt: Configuration
      mask DialogControl ContFaultABC Prompt: Fault :
      mask DialogControl ContBreakerParam Prompt: Breaker parameters :
      mask DialogControl ContZeroCross Prompt: Control initial voltage phase of first fault
      mask DialogControl Container5 Prompt: Arc Parameters
      mask DialogControl ContArcParam Prompt: Arc fault parameters
      mask DialogControl ContArcVoltage Prompt: Arc Ignition Voltage
      mask DialogControl ContArcLim Prompt: Arc limitations
      mask DialogControl ContFilterPetSlep Prompt: Filtering
      mask DialogControl ContInterruption Prompt: Interruption
      mask DialogControl Container14 Prompt: Settings for different types of fault interruption
      mask Display:
      | % port_label('input',1,'Iabc');
      | 
      | port_label('lconn',1,'A');
      | port_label('lconn',2,'B');
      | port_label('lconn',3,'C');
      | 
      | disp('   SPGF    ');
  meas : Subsystem
  A : PMIOPort  Side=Left
  B : PMIOPort  Port=2  Side=Left
  C : PMIOPort  Port=3  Side=Left
  connections:
  meas/LConn3 -- C/RConn1
  meas/LConn1 -- A/RConn1
  meas/LConn2 -- B/RConn1
  fault/LConn3 -- meas/RConn3
  fault/LConn2 -- meas/RConn2
  fault/LConn1 -- meas/RConn1

== system SPGF_FSK_0000_R2022b/TP11 ==
  Load : spsThreePhaseParallelRLCLoadLib/Three-Phase Parallel RLC Load  Commented=on  LConnTagsString=A|B|C  Configuration=Y (grounded)  NominalVoltage=380  Vabc=[1e3 1e3 1e3]  Vabcp=[1e3 1e3 1e3]  NominalFrequency=50  UnbalancedPower=off  ActivePower=896000/2  InductivePower=403200/2  CapacitivePower=0  Pabc=[10e3 9e3 11e3]  QLabc=[100 90 110]  QCabc=[100 90 110]  Pabcp=[10e3 9e3 11e3]  QLabcp=[100 90 110]  QCabcp=[100 90 110]  Measurements=None  LoadType=constant PQ
  Nonlinear Load : Subsystem  Commented=on
  Nonlinear Load 3ph : Subsystem
  Q : Subsystem
  T : spsThreePhaseTransformerTwoWindingsLib/Three-Phase Transformer (Two Windings)  Winding1Connection=Y  Winding2Connection=Yg  CoreType=Three single-phase transformers  SetSaturation=on  Hysteresis=off  DataFile='hysteresis'  SetInitialFlux=off  Measurements=None  UNITS=pu  NominalPower=[800000, 50]  Winding1=[10250, 0.00562500, 0.03250000]  Winding2=[400.00, 0.00562500, 0.03250000]  Rm=680.851  Lm=76.9231  L0=2  Saturation=[0 0;0.01774 0.324129;0.0487637 0.61284;0.0980856 0.825118;0.2 1;0.309543 1.08024;0.652348 1.17344;2.0357 1.26115;6.0215 1.36094;12.4388 1.49469]  InitialFluxes=[0.0304364546455999 0.882164054946781 -0.912600509593102]  BreakLoop=on  DiscreteSolver=Trapezoidal iterative  DataType=off  TransfoNumber=1
  Three-Phase Series RLC Load : spsThreePhaseSeriesRLCLoadLib/Three-Phase Series RLC Load  Commented=on  LConnTagsString=A|B|C  Configuration=Y (grounded)  NominalVoltage=380  Vabc=[1e3 1e3 1e3]  Vabcp=[1e3 1e3 1e3]  NominalFrequency=50  UnbalancedPower=off  ActivePower=896000/2  InductivePower=403200/2  CapacitivePower=0  Pabc=[10e3 9e3 11e3]  QLabc=[100 90 110]  QCabc=[100 90 110]  Pabcp=[10e3 9e3 11e3]  QLabcp=[100 90 110]  QCabcp=[100 90 110]  Measurements=None  LoadType=constant Z
  Three-Phase Series RLC Load1 : spsThreePhaseSeriesRLCLoadLib/Three-Phase Series RLC Load  LConnTagsString=A|B|C  Configuration=Y (grounded)  NominalVoltage=380  Vabc=[1e3 1e3 1e3]  Vabcp=[1e3 1e3 1e3]  NominalFrequency=50  UnbalancedPower=off  ActivePower=0.1*896000/2  InductivePower=0  CapacitivePower=0  Pabc=[10e3 9e3 11e3]  QLabc=[100 90 110]  QCabc=[100 90 110]  Pabcp=[10e3 9e3 11e3]  QLabcp=[100 90 110]  QCabcp=[100 90 110]  Measurements=None  LoadType=constant Z
  Three-Phase Series RLC Load2 : spsThreePhaseSeriesRLCLoadLib/Three-Phase Series RLC Load  LConnTagsString=A|B|C  Configuration=Y (grounded)  NominalVoltage=380  Vabc=[1e3 1e3 1e3]  Vabcp=[1e3 1e3 1e3]  NominalFrequency=50  UnbalancedPower=off  ActivePower=0.9*896000/2  InductivePower=403200/2  CapacitivePower=0  Pabc=[10e3 9e3 11e3]  QLabc=[100 90 110]  QCabc=[100 90 110]  Pabcp=[10e3 9e3 11e3]  QLabcp=[100 90 110]  QCabcp=[100 90 110]  Measurements=None  LoadType=constant Z
  A : PMIOPort  Side=Right
  B : PMIOPort  Port=2  Side=Right
  C : PMIOPort  Port=3  Side=Right
  connections:
  Q/RConn2 -- B/RConn1
  Q/RConn1 -- A/RConn1
  Q/RConn3 -- C/RConn1
  Q/LConn1 -- T/LConn1
  Q/LConn2 -- T/LConn2
  Q/LConn3 -- T/LConn3
  Load/LConn2 -- Three-Phase Series RLC Load1/LConn2 -- Three-Phase Series RLC Load2/LConn2 -- Three-Phase Series RLC Load/LConn2 -- Nonlinear Load 3ph/LConn2 -- Nonlinear Load/LConn2 -- T/RConn2
  Load/LConn1 -- Three-Phase Series RLC Load1/LConn1 -- Three-Phase Series RLC Load2/LConn1 -- Three-Phase Series RLC Load/LConn1 -- Nonlinear Load 3ph/LConn1 -- Nonlinear Load/LConn1 -- T/RConn1
  Load/LConn3 -- Three-Phase Series RLC Load1/LConn3 -- Three-Phase Series RLC Load2/LConn3 -- Three-Phase Series RLC Load/LConn3 -- Nonlinear Load 3ph/LConn3 -- Nonlinear Load/LConn3 -- T/RConn3
